simulink model "MassepunktAufSchieferEbene"  (Simulink 7.1)
settings: Solver=ode45  StartTime=0.0  StopTime=10.0  RelTol=1e-3
settings Model: Creator=Meisel  LastModifiedBy=Meisel

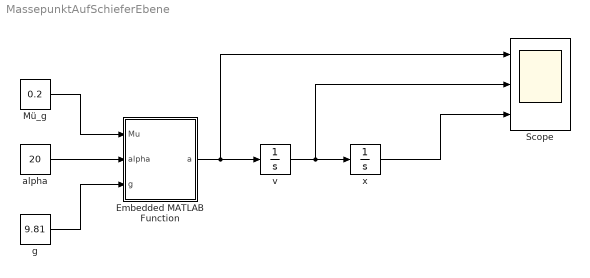
== system MassepunktAufSchieferEbene ==
  Embedded MATLAB Function : Stateflow chart
  Mü_g : Constant  Value=0.2  OutDataType=sfix(16)  OutScaling=2^0
  Scope : Scope  NumInputPorts=3
      settings: YMin=-5~-5~-5  YMax=5~5~5
  alpha : Constant  Value=20  OutDataType=sfix(16)  OutScaling=2^0
  g : Constant  Value=9.81  OutDataType=sfix(16)  OutScaling=2^0
  v : Integrator
  x : Integrator
  wires:
  v/1 -> x/1, Scope/2
  Embedded MATLAB Function/1(a) -> v/1, Scope/1
  alpha/1 -> Embedded MATLAB Function/2(alpha)
  Mü_g/1 -> Embedded MATLAB Function/1(Mu)
  g/1 -> Embedded MATLAB Function/3(g)
  x/1 -> Scope/3

== matlab function Embedded MATLAB Function ==
  data: Mu input double; a output double; alpha input double; g input double
function a = fcn(Mu, alpha, g)
% This block supports the Embedded MATLAB subset.
% See the help menu for details. 
alpha_Bogen=alpha*pi/180;
a = g*(sin(alpha_Bogen) - Mu*cos(alpha_Bogen));
